simulink library "cart2sph_degas"  (R2018b)
settings: Solver=VariableStepAuto  StartTime=0.0  StopTime=10.0  RelTol=1e-3
settings Model: Creator=BI28030  LastModifiedBy=BI28030

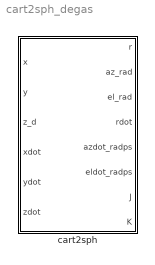
== system cart2sph_degas ==
  cart2sph : MATLAB Function  TreatAsAtomicUnit=on

== matlab function cart2sph_degas/cart2sph ==
  data: x input; r output; az_rad output; el_rad output; rdot output; azdot_radps output; eldot_radps output; y input; z_d input; J output; xdot input; ydot input; zdot input; K output
function [r,az_rad,el_rad,rdot,azdot_radps,eldot_radps,J,K] = cartesian2spherical(x, y, z_d, xdot, ydot, zdot)
%Convert North, East, Down coordinates to Range, Azimuth, Elevation
% Returns the Jacobian J of the 3x3 transformation and the off-diagonal
% Jacobian block K for the 6x6 transformation (so J' = [J zeros(3); K J])

% range
xyz = [ x; y; z_d ];
r = norm(xyz);

% azimuth and azimuth rate
az_rad = atan2(y,x);

% elevation and elevation rate
el_rad = asin(-z_d/r);

% Jacobian (r,az,el)/(x,y,z)
h = norm( [ x y ] );
J = [       xyz'/r; ...
      -y/h^2      x/h^2        0; ...
      x*z_d/(h*r^2) y*z_d/(h*r^2) -h/r^2 ];

% d(r,za,el)/dt = J * d(x,y,z)/dt
rdot = J(1,:) * [xdot; ydot; zdot];
azdot_radps = J(2,:) * [xdot; ydot; zdot];
eldot_radps = J(3,:) * [xdot; ydot; zdot];
  
% position-velocity correlations (copied from sph->cart, get inverse of that K with Schur complement)
Kxdot_r = -(y/r)*azdot_radps + (z_d/r)*cos(az_rad)*eldot_radps;
Kxdot_az = -rdot*(y/r) - x*azdot_radps - z_d*sin(az_rad)*eldot_radps;
Kxdot_el = rdot*(z_d/r)*cos(az_rad) - z_d*sin(az_rad)*azdot_radps - x*eldot_radps;

Kydot_r = (z_d/r)*sin(az_rad)*eldot_radps + (x/r)*azdot_radps;
Kydot_az = rdot*(x/r) + z_d*cos(az_rad)*eldot_radps - y*azdot_radps;
Kydot_el = rdot*(z_d/r)*sin(az_rad) - y*eldot_radps + z_d*cos(az_rad)*azdot_radps;

Kzdot_r = -cos(el_rad)*eldot_radps;
Kzdot_az = 0;
Kzdot_el = -rdot*cos(el_rad) - z_d*eldot_radps;

K = -J*[ Kxdot_r   Kxdot_az   Kxdot_el;
         Kydot_r   Kydot_az   Kydot_el;
         Kzdot_r   Kzdot_az   Kzdot_el   ]*J;
